simulink model "Complete_HPP_Model_PEM_WIndTurbine"  (R2022a)
settings: Solver=ode4  StartTime=0.0  StopTime=5  FixedStep=1e-6  MaxStep=50e-7  RelTol=1e-3
undefined symbols (not defined in the file or in its folder): DiscIntNeverNeededParam, Ts_Control
libraries: spsMeanLib x9, spsSeriesRLCBranchLib x8, spsIGBTDiodeLib x7, spsVoltageMeasurementLib x6, spsThreePhaseVIMeasurementLib x4, spsDiodeLib x4, spsCurrentMeasurementLib x4, spsMosfetLib x3, spsThreePhaseSeriesRLCBranchLib x2, spsGroundLib x2, spsSawtoothGeneratorLib x2, spsWindTurbineLib x1
(part 1 of 2)
settings Model: Creator=TASOS  LastModifiedBy=nikos
settings DebuggingCC: AlgebraicLoopMsg=none

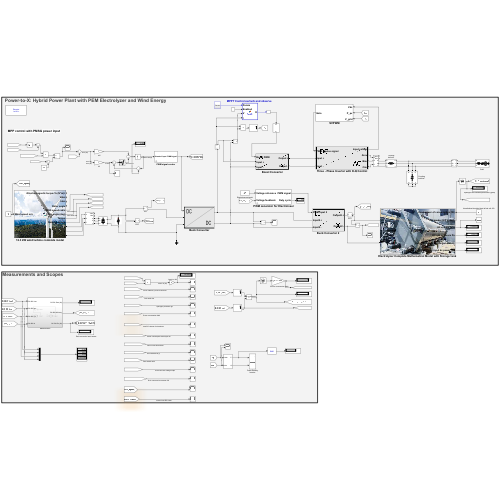
[thumbnail: Simulink's stored preview of the top-level diagram]
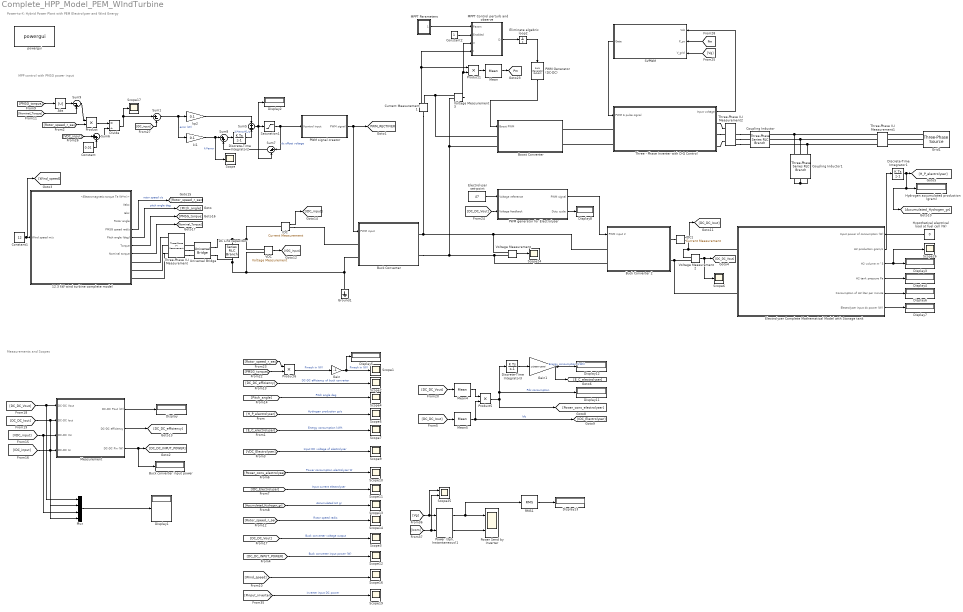
== system Complete_HPP_Model_PEM_WIndTurbine ==
  note: Power-to-X: Hybrid Power Plant with PEM Electrolyzer and Wind Energy
  note: Measurements and Scopes
  note: MPP control with PMSG power input
  12.3 kW wind turbine complete model : Subsystem  mask{Nominal_mechanical_output_power=12.3e3, R=1.3, Base_wind=12}
      mask prompts: Nominal_mechanical_output_power "Nominal_mechanical_output_power (W)"; R "Rotor radiance (m)"; Base_wind "Base_wind (m/s)"
      mask Display: image('$imagefile'); % Use "Edit Image" on toolstrip to change.
  Abs : Abs  SaturateOnIntegerOverflow=off
  Boost Converter : Subsystem
      mask Display: image('$imagefile'); % Use "Edit Image" on toolstrip to change.
  Buck Converter : Subsystem
      mask Display: image('$imagefile'); % Use "Edit Image" on toolstrip to change.
  "Buck Converter 2 " : Subsystem
      mask Display: image('$imagefile'); % Use "Edit Image" on toolstrip to change.
  Buck converter input power : Display
  Constant : Constant  Value=0.01
  Constant1 : Constant  Value=12
  Constant2 : Constant
  Coupling Inductor : spsThreePhaseSeriesRLCBranchLib/Three-Phase Series RLC Branch  LConnTagsString=A|B|C  RConnTagsString=A|B|C  BranchType=L  Resistance=0.09  Inductance=15e-3  Capacitance=1e-6  Measurements=None
  Coupling Inductor1 : spsThreePhaseSeriesRLCBranchLib/Three-Phase Series RLC Branch  LConnTagsString=A|B|C  RConnTagsString=A|B|C  BranchType=C  Resistance=0.09  Inductance=0.28e-3  Capacitance=3e-6  Measurements=None
  Current Measurement1 : spsCurrentMeasurementLib/Current Measurement  PhasorSimulation=off  OutputType=Complex  PSBequivalent=0
  DC Link capacitor : spsSeriesRLCBranchLib/Series RLC Branch  LConnTagsString=__new0  RConnTagsString=__new0  BranchType=C  Resistance=0.005  Inductance=200e-6  SetiL0=off  InitialCurrent=0  Capacitance=3600e-6  Setx0=off  InitialVoltage=150  Measurements=None
  Discrete-Time Integrator1 : DiscreteIntegrator  SampleTime=1e-6  ICPrevOutput=DiscIntNeverNeededParam  ICPrevScaledInput=DiscIntNeverNeededParam
  Discrete-Time Integrator2 : DiscreteIntegrator  InitialCondition=0.01  SampleTime=1e-6  LimitOutput=on  UpperSaturationLimit=0.9  LowerSaturationLimit=0.01  ICPrevOutput=DiscIntNeverNeededParam  ICPrevScaledInput=DiscIntNeverNeededParam
  Discrete-Time Integrator3 : DiscreteIntegrator  SampleTime=1e-6  ICPrevOutput=DiscIntNeverNeededParam  ICPrevScaledInput=DiscIntNeverNeededParam
  Display{,1..8,11..13} (12 alike) : Display
  Divide : Product  Inputs=*/
  Electrolyser set-point : Constant  Value=47
  "Electrolyzer Complete Mathematical Model with Storage tank " : Subsystem
      settings: PortSchema="{\"entries\":[{\"content\":{\"sides\":[{\"content\":{\"connectorIds\":[\"In1\",\"Out1\",\"Out2\",\"Out3\",\"Out4\",\"Out5\"]},\"type\":\"ConnectorPlacement.EquallySpacedRectSide\",\"uuid\":\"586e2a01-0b83-4db1-b05b-c9425d179327\"},{\"content\":{\"connectorIds\":[\"RConn1\",\"RConn2\"],\"side\":\"RIGHT\"},\"type\":\"ConnectorPlacement.EquallySpacedRectSide\",\"uuid\":\"98998693-1c1d-43a0-8265-c06eb7552525\"},{\"content\":{\"connectorIds\":[],\"side\":\"TOP\"},\"type\":\"ConnectorPlacement.EquallySpacedRectSide\",\"uuid\":\"57c96d85-f297-491e-8250-1f4aa33eee63\"}]},\"type\":\"ConnectorPlacement.EquallySpacedConnector\",\"uuid\":\"2efb03bc-2da9-4118-9dbe-8a463fcc009b\"}],\"packageUris\":[\"http://schema.mathworks.com/mf0/Connector/R2020b\"],\"version\":\"1.0\"}"
      mask Display: image('$imagefile'); % Use "Edit Image" on toolstrip to change.
  Eliminate algebric loop2 : UnitDelay  InitialCondition=0.485  SampleTime=Ts_Control  HasFrameUpgradeWarning=on
  Gain : Gain  Gain=-1
  Gain1 : Gain  Gain=1/(3600*1000)
  Grid1 : spsThreePhaseSourceLib/Three-Phase Source  InternalConnection=Yg  VoltagePhases=off  Voltage=400  PhaseAngle=0  Voltage_phases=[25e3 25e3 25e3]/sqrt(3)  PhaseAngles_phases=[0 -120 +120]  Frequency=50  NonIdealSource=on  SpecifyImpedance=on  Resistance=0.8929  Inductance=16.58e-3  ShortCircuitLevel=100e6  BaseVoltage=400  XRratio=10  BusType=swing  Pref=0  Qref=0  Prefabc=[10e3, 10e3, 10e3]  Qrefabc=[0, 0, 0]  Qmin=-inf  Qmax=inf
  Ground1 : spsGroundLib/Ground  LConnTagsString=a
  Hydrogen accumulated production (gram) : Display
  Hypothetical electrical load at fuel cell (W) : Constant  Value=0
  IDC : spsCurrentMeasurementLib/Current Measurement  PhasorSimulation=off  OutputType=Complex  PSBequivalent=0
  IDC1 : spsCurrentMeasurementLib/Current Measurement  PhasorSimulation=off  OutputType=Complex  PSBequivalent=0
  MPPT Parameters : Subsystem
  "MPPT Control perturb and observe  " : MATLAB Function  TreatAsAtomicUnit=on
  Mean : spsMeanLib/Mean  Freq=50  Vinit=0  Ts=0
  Mean4 : spsMeanLib/Mean  Freq=50  Vinit=0  Ts=1e-6
  Mean5 : spsMeanLib/Mean  Freq=50  Vinit=0  Ts=1e-6
  Measurement : Subsystem
  Mux : Mux
  PWM Generator (DC-DC) : spsPWMGeneratorDCDCLib/PWM Generator (DC-DC)  Fsw=10000  Ts=0
  PWM generator for Electrolyser : Subsystem  mask{fs=20000, ki2=0.005, kp2=0.05}
      mask prompts: fs "Switching frequency"; ki2 "ki"; kp2 "kp"
  PWM signal creator : Subsystem  mask{Fs=10e3, Ts=0}
      mask prompts: Fs "Switching frequency"; Ts "Sample time"
  "Power (3ph, Instantaneous)1" : spsPower3phInstantaneousLib/Power (3ph, Instantaneous)
  Power Send by Inverter : Scope  NumInputPorts=2
  Product{,1,5..6} (4 alike) : Product
  RMS1 : spsRMSLib/RMS  TrueRMS=on  Freq=60  RMSInit=120  Ts=0
  SVPWM : Subsystem
  Saturation1 : Saturate  UpperLimit=0.9  LowerLimit=0
  Scope{,1..7,9..14,17,19,24,26} (18 alike) : Scope
  Scope16 : Scope  NumInputPorts=2
  Scope25 : Scope  NumInputPorts=2
  Sum1 : Sum  Inputs=|+-
  Sum5 : Sum
  Sum6 : Sum  Inputs=|++
  Sum7 : Sum  Inputs=|+-
  Sum8 : Sum  Inputs=|++
  Sum9 : Sum  Inputs=|-+
  Three - Phase Inverter with D-Q Control : Subsystem
      mask Display: image('$imagefile'); % Use "Edit Image" on toolstrip to change.
  Three-Phase V-I Measurement : spsThreePhaseVIMeasurementLib/Three-Phase V-I Measurement  VoltageMeasurement=phase-to-ground  SetLabelV=off  LabelV=Vabc  Vpu=off  VpuLL=off  CurrentMeasurement=yes  SetLabelI=off  LabelI=Iabc  Ipu=off  Pbase=100e6  Vbase=500e3  OutputType=Complex  PhasorSimulation=off  PSBequivalent=0
  Three-Phase V-I Measurement1 : spsThreePhaseVIMeasurementLib/Three-Phase V-I Measurement  VoltageMeasurement=phase-to-ground  SetLabelV=on  LabelV=Vg  Vpu=off  VpuLL=off  CurrentMeasurement=yes  SetLabelI=on  LabelI=Icom  Ipu=off  Pbase=100e6  Vbase=500e3  OutputType=Complex  PhasorSimulation=off  PSBequivalent=0
  Three-Phase V-I Measurement2 : spsThreePhaseVIMeasurementLib/Three-Phase V-I Measurement  VoltageMeasurement=phase-to-phase  SetLabelV=off  LabelV=Vg  Vpu=off  VpuLL=off  CurrentMeasurement=yes  SetLabelI=off  LabelI=Icom  Ipu=off  Pbase=100e6  Vbase=500e3  OutputType=Complex  PhasorSimulation=off  PSBequivalent=0
  Universal Bridge : spsUniversalBridgeLib/Universal Bridge  Arms=3  SnubberResistance=1e6  SnubberCapacitance=inf  Device=Diodes  Ron=1e-3  Lon=0  ForwardVoltages="[  0  0  ]"  ForwardVoltage=0  GTOparameters=[ 10e-6 , 20e-6 ]  IGBTparameters=[ 1e-6 , 2e-6 ]  Measurements=None  Measurements_2=None  converterType=Rectifier
  VDC : spsVoltageMeasurementLib/Voltage Measurement  PhasorSimulation=off  OutputType=Complex  PSBequivalent=0
  Voltage Measurement : spsVoltageMeasurementLib/Voltage Measurement  PhasorSimulation=off  OutputType=Complex  PSBequivalent=0
  Voltage Measurement2 : spsVoltageMeasurementLib/Voltage Measurement  PhasorSimulation=off  OutputType=Complex  PSBequivalent=0
  Voltage Measurement3 : spsVoltageMeasurementLib/Voltage Measurement  PhasorSimulation=off  OutputType=Complex  PSBequivalent=0
  ki1 : Gain  Gain=0.1
  kp2 : Gain  Gain=0.1
  powergui : spspowerguiLib/powergui  Priority=1  SimulationMode=Discrete  SampleTime=1e-6  frequency=60  Iterations=50  frequencyindice=0  Pbase=100e6  ErrMax=1e-4  UnitsV=kV  UnitsW=MW  buscounter=0  FunctionMessages=off  echomessages=off  EnableUseOfTLC=off  CurrentSourceSwitches=off  DisableSnubberDevices=off  DisableRonSwitches=off  DisableVfSwitches=off  DisplayEquations=off  AutomaticDiscreteSolvers=off  SolverType=Tustin/Backward Euler (TBE)  Interpol=off  ExternalGateDelay=off  methode=off  Ts=100  x0status=blocks  SPID=on  SwTol=0  HookPort=off  NonlinearTolerance=1e-4  nMaxIteration=100  ContinueOnMaxIteration=off  RestoreLinks=warning  ResistiveCurrentMeasurement=off  Frange=[0:2:500]  Ylog=off  Xlog=on  ShowGrid=off  save=off  variable=ZData  structure=0  ZoomFFT=off  StartTime=0.0  cycles=1  DisplayStyle=1  fundamental=60  FreqAxis=off  MaxFrequency=1000  frequencyindicesteady=1  RmsSteady=1  display=off
  tag scope: PWM_RECTIFIER=global, Pm=global
  wires:
  Mean5/1 -> Product5/2, [IDC_Electrolyser]  "Idc"
  Discrete-Time Integrator3/1 -> Gain1/1
  Gain1/1 -> [E_C_electrolyser], Display12/1  "Energy consumption (kWh)"
  Product5/1 -> Discrete-Time Integrator3/1, Display11/1, [Power_cons_electrolyser]  "Pdc consumption"
  Mean4/1 -> Product5/1
  Product6/1 -> Gain/1  "Pmech in (W)"
  [DC_DC_efficiency] -> Scope2/1  "DC-DC efficiency of buck converter"
  [Pitch_angle] -> Scope4/1  "Pitch angle deg"
  [E_C_electrolyser] -> Scope7/1  "Energy consumption kWh"
  [IDC_Electrolyser] -> Scope11/1  "Input current electrolyser"
  [H_P_electrolyser] -> Scope5/1  "Hydrogen production gr/s"
  [Accumulated_Hydrogen_gr] -> Scope13/1  "Accumulated H2 gr"
  [Power_cons_electrolyser] -> Scope10/1  "Power consumption electrolyser W"
  [VDC_Electrolyser] -> Scope9/1  "Input DC voltage of electrolyser"
  12.3 kW wind turbine complete model/6(Pitch angle (deg)) -> [Pitch_angle]  "pitch angle deg"
  12.3 kW wind turbine complete model/5(PMSG speed rad/s) -> [Rotor_speed_r_sec]  "rotor speed r/s"
  Gain/1 -> Scope1/1, Display5/1  "Pmech in (W)"
  [Rotor_speed_r_sec] -> Scope14/1  "Rotor speed rad/s"
  [DC_DC_Vout] -> Scope3/1  "Buck converter voltage output"
  IDC1/1 -> [DC_DC_Iout]
  Measurement/1(DC-DC Pout (W)) -> Display/1
  [DC_DC_Vout] -> Mux/1, Measurement/1(DC-DC Vout)
  [DC_DC_Iout] -> Mux/2, Measurement/2(DC-DC Iout)
  [VDC_input] -> Mux/3, Measurement/3(DC-DC Vin)
  [IDC_input] -> Mux/4, Measurement/4(DC-DC Iin)
  Measurement/2(DC-DC efficiency) -> [DC_DC_efficiency]
  Measurement/3(DC-DC Pin (W)) -> Buck converter input power/1, [DC_DC_INPUT_POWER]
  [DC_DC_INPUT_POWER] -> Scope12/1  "Buck converter input power (W)"
  Mux/1 -> Display1/1
  [DC_DC_Vout] -> Mean4/1
  [DC_DC_Iout] -> Mean5/1
  [PMSG_torque] -> Product6/2
  [Rotor_speed_r_sec] -> Product6/1
  [Wind_speed] -> Scope16/2
  VDC/1 -> [VDC_input]
  IDC/1 -> [IDC_input]
  Constant1/1 -> 12.3 kW wind turbine complete model/1(Wind speed m/s), [Wind_speed]
  Discrete-Time Integrator1/1 -> [H_P_electrolyser], Hydrogen accumulated production (gram)/1, [Accumulated_Hydrogen_gr]
  "Electrolyzer Complete Mathematical Model with Storage tank "/1(H2 production gram/s) -> Discrete-Time Integrator1/1
  [Pinput_inverter] -> Scope19/1  "inverter input DC power"
  "Electrolyzer Complete Mathematical Model with Storage tank "/2(H2 volume m^3) -> Display3/1, Scope26/1
  "Electrolyzer Complete Mathematical Model with Storage tank "/3(H2 tank pressure Pa) -> Display4/1
  Hypothetical electrical load at fuel cell (W)/1 -> "Electrolyzer Complete Mathematical Model with Storage tank "/1(Input power of consumption (W))
  "Electrolyzer Complete Mathematical Model with Storage tank "/4(Consumption of H2 liter per minute) -> Display6/1
  "Electrolyzer Complete Mathematical Model with Storage tank "/5(Electrolyser input dc power (W)) -> Display7/1
  Voltage Measurement2/1 -> [DC_DC_Vout], Scope6/1
  Electrolyser set-point/1 -> PWM generator for Electrolyser/1(Voltage reference)
  [DC_DC_Vout] -> PWM generator for Electrolyser/2(Voltage feedback)
  PWM generator for Electrolyser/2(Duty cycle) -> Display8/1
  Voltage Measurement/1 -> Scope24/1
  12.3 kW wind turbine complete model/7(Torque) -> [PMSG_torque]
  12.3 kW wind turbine complete model/8(Nominal torque) -> [Nominal_Torque]
  PWM signal creator/1(PWM signal) -> [PWM_RECTIFIER], Buck Converter/1(PWM input)
  PWM generator for Electrolyser/1(PWM signal) -> "Buck Converter 2 "/1(PWM input 2)
  [Pm] -> SVPWM/2(P_pv)
  [Vg] -> SVPWM/3(V_grid)
  MPPT Parameters/1(Param) -> "MPPT Control perturb and observe  "/1(Param)
  Mean/1 -> [Pm]
  Eliminate algebric loop2/1 -> PWM Generator (DC-DC)/1
  "MPPT Control perturb and observe  "/1(D) -> Eliminate algebric loop2/1
  Constant2/1 -> "MPPT Control perturb and observe  "/2(Enabled)
  Product1/1 -> Mean/1
  Current Measurement1/1 -> Product1/1, "MPPT Control perturb and observe  "/4(I)
  Voltage Measurement3/1 -> Product1/2, "MPPT Control perturb and observe  "/3(V)
  PWM Generator (DC-DC)/1 -> Boost Converter/1(Boost PWM)
  Three - Phase Inverter with D-Q Control/1(Input voltage) -> SVPWM/1(Vdc)
  SVPWM/1(Gate) -> Three - Phase Inverter with D-Q Control/1(PWM 6 pulse signal)
  Sum8/1 -> Discrete-Time Integrator2/1
  [IDC_input] -> Sum1/2
  ki1/1 -> Sum8/1, Scope/1  "ki*error"
  Discrete-Time Integrator2/1 -> Sum5/2  "ki*error*1/s"
  Abs/1 -> Sum9/1
  Sum5/1 -> Sum7/2, Display2/1, Saturation1/1
  Divide/1 -> Sum1/1, Scope17/1
  Sum7/1 -> Sum8/2
  Sum9/1 -> Product/1
  Saturation1/1 -> PWM signal creator/1("Vcontrol input "), Sum7/1  "dc offset voltage"
  Product/1 -> Divide/1
  [VDC_input] -> Sum6/1
  Sum1/1 -> kp2/1, ki1/1  "error (W)"
  kp2/1 -> Sum5/1
  [Nominal_Torque] -> Sum9/2
  [Rotor_speed_r_sec] -> Product/2
  Sum6/1 -> Divide/2
  [PMSG_torque] -> Abs/1
  Constant/1 -> Sum6/2
  "Power (3ph, Instantaneous)1"/2 -> Power Send by Inverter/2
  "Power (3ph, Instantaneous)1"/1 -> RMS1/1, Power Send by Inverter/1
  [Vg] -> Scope25/1, "Power (3ph, Instantaneous)1"/1
  [Icom] -> Scope25/2, "Power (3ph, Instantaneous)1"/2
  RMS1/1 -> Display13/1
  connections:
  DC Link capacitor/LConn1 -- IDC/LConn1 -- VDC/LConn1 -- Universal Bridge/RConn1
  Universal Bridge/LConn1 -- Three-Phase V-I Measurement/RConn1
  Three-Phase V-I Measurement/RConn2 -- Universal Bridge/LConn2
  Three-Phase V-I Measurement/RConn3 -- Universal Bridge/LConn3
  Three-Phase V-I Measurement/LConn1 -- 12.3 kW wind turbine complete model/RConn1
  Three-Phase V-I Measurement/LConn2 -- 12.3 kW wind turbine complete model/RConn2
  Three-Phase V-I Measurement/LConn3 -- 12.3 kW wind turbine complete model/RConn3
  IDC1/RConn1 -- "Electrolyzer Complete Mathematical Model with Storage tank "/RConn1 -- Voltage Measurement2/LConn1
  Voltage Measurement/LConn1 -- "Buck Converter 2 "/LConn1 -- Current Measurement1/LConn1 -- Buck Converter/RConn1
  IDC/RConn1 -- Buck Converter/LConn1
  VDC/LConn2 -- Ground1/LConn1 -- Buck Converter/LConn2 -- Universal Bridge/RConn2 -- DC Link capacitor/RConn1
  Voltage Measurement/LConn2 -- Voltage Measurement3/LConn2 -- Boost Converter/LConn2 -- Buck Converter/RConn2 -- "Buck Converter 2 "/LConn2
  Voltage Measurement2/LConn2 -- "Buck Converter 2 "/RConn2 -- "Electrolyzer Complete Mathematical Model with Storage tank "/RConn2
  "Buck Converter 2 "/RConn1 -- IDC1/LConn1
  Current Measurement1/RConn1 -- Boost Converter/LConn1 -- Voltage Measurement3/LConn1
  Grid1/RConn1 -- Three-Phase V-I Measurement1/RConn1
  Three-Phase V-I Measurement1/LConn1 -- Coupling Inductor1/LConn1 -- Coupling Inductor/RConn1
  Grid1/RConn3 -- Three-Phase V-I Measurement1/RConn3
  Grid1/RConn2 -- Three-Phase V-I Measurement1/RConn2
  Three-Phase V-I Measurement1/LConn2 -- Coupling Inductor1/LConn2 -- Coupling Inductor/RConn2
  Three-Phase V-I Measurement1/LConn3 -- Coupling Inductor1/LConn3 -- Coupling Inductor/RConn3
  Coupling Inductor1/RConn1 -- Coupling Inductor1/RConn3 -- Coupling Inductor1/RConn2
  Three - Phase Inverter with D-Q Control/LConn1 -- Boost Converter/RConn1
  Three - Phase Inverter with D-Q Control/LConn2 -- Boost Converter/RConn2
  Three - Phase Inverter with D-Q Control/RConn1 -- Three-Phase V-I Measurement2/LConn1
  Three - Phase Inverter with D-Q Control/RConn2 -- Three-Phase V-I Measurement2/LConn2
  Three - Phase Inverter with D-Q Control/RConn3 -- Three-Phase V-I Measurement2/LConn3
  Three-Phase V-I Measurement2/RConn1 -- Coupling Inductor/LConn1
  Three-Phase V-I Measurement2/RConn2 -- Coupling Inductor/LConn2
  Three-Phase V-I Measurement2/RConn3 -- Coupling Inductor/LConn3

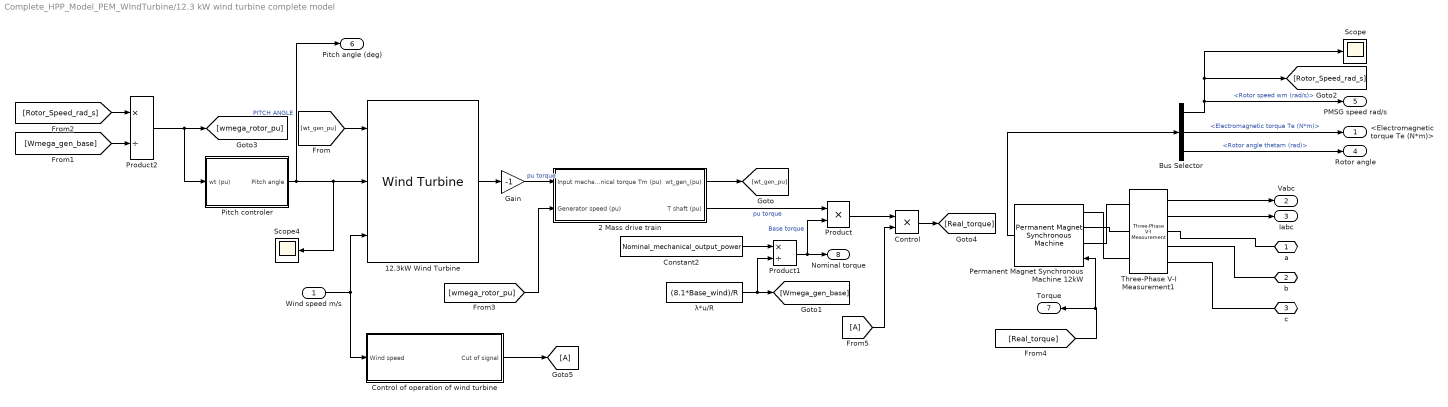
== system Complete_HPP_Model_PEM_WIndTurbine/12.3 kW wind turbine complete model ==
  Wind speed m/s : Inport
  12.3kW Wind Turbine : spsWindTurbineLib/Wind Turbine  Pnom=Nominal_mechanical_output_power  Pelec_base=Nominal_mechanical_output_power/0.9  wind_base=Base_wind  P_wind_base=0.85  speed_nom=1.2  pitch_angle=0  c1_c6="[0.51763          116          0.4            5           21     0.006795]"  cp_nom=0.48  lambda_nom=8.1
      link override Gain: Gain=-1
      settings: SourceProductBaseCode=PS
  2 Mass drive train : Subsystem  mask{H=4, w_base=(8.1*Base_wind)/R, shaft_stiffness=0.3, Ts=1e-6}
      mask prompts: H "Input H"; w_base "Input w base"; shaft_stiffness "Input shaft stiffness"; Ts "Sample time (s)"
  Bus Selector : BusSelector  OutputSignals=Rotor speed wm (rad/s),Electromagnetic torque Te (N*m),Rotor angle thetam (rad)
  Constant2 : Constant  Value=Nominal_mechanical_output_power
  Control : Product
  Control of operation of wind turbine : Subsystem
  From5 : From
  Gain : Gain  Gain=-1
  Goto5 : Goto
  Permanent Magnet Synchronous Machine 12kW : spsPermanentMagnetSynchronousMachineLib/Permanent Magnet Synchronous Machine  NbPhases=3  FluxDistribution=Sinusoidal  RotorType=Salient-pole  MechanicalLoad=Torque Tm  PresetModel=No  ShowDetailedParameters=on  MeasurementBus=off  Resistance=0.425  Inductance=8.5e-3  dqInductances=[0.835e-3, 0.835e-3]  La=1.975e-07  MachineConstant=Flux linkage established by magnets (V.s)  Flux=0.5333  VoltageCst=483.6496  TorqueCst=3.9997  Flat=120  Mechanical=[0.0027 0.000303448 5]  PolePairs=4  InitialConditions=[0,0, 0,0]  InitialConditions5ph=[0 0 0 0 0 0]  RefAngle=90 degrees behind phase A axis (modified Park)  IterativeDiscreteModel=Trapezoidal non iterative  TsBlock=-1  TsPowergui=0
  Pitch controler : Subsystem  mask{Ki=10, Kp=1000}
  Product : Product  Inputs=**
  Product1 : Product  Inputs=*/
  Product2 : Product  Inputs=*/
  Scope : Scope
  Scope4 : Scope
  Three-Phase V-I Measurement1 : spsThreePhaseVIMeasurementLib/Three-Phase V-I Measurement  VoltageMeasurement=phase-to-phase  SetLabelV=off  LabelV=Vabc  Vpu=off  VpuLL=off  CurrentMeasurement=yes  SetLabelI=off  LabelI=Iabc  Ipu=off  Pbase=100e6  Vbase=500e3  OutputType=Complex  PhasorSimulation=off  PSBequivalent=0
  λ*u/R : Constant  Value=(8.1*Base_wind)/R
  a : PMIOPort  Side=Right
  b : PMIOPort  Port=2  Side=Right
  c : PMIOPort  Port=3  Side=Right
  <Electromagnetic torque Te (N*m)> : Outport
  Vabc : Outport  Port=2
  Iabc : Outport  Port=3
  Rotor angle : Outport  Port=4
  PMSG speed rad/s : Outport  Port=5
  Pitch angle (deg) : Outport  Port=6
  Torque : Outport  Port=7
  Nominal torque : Outport  Port=8
  wires:
  Pitch controler/1(Pitch angle) -> Pitch angle (deg)/1, Scope4/1, 12.3kW Wind Turbine/2  "PITCH ANGLE"
  Product2/1 -> [wmega_rotor_pu], Pitch controler/1(wt (pu))
  [wmega_rotor_pu] -> 2 Mass drive train/2(Generator speed (pu))
  Bus Selector/1 -> Scope/1, [Rotor_Speed_rad_s], PMSG speed rad/s/1  "<Rotor speed wm (rad/s)>"
  [Rotor_Speed_rad_s] -> Product2/1
  λ*u/R/1 -> [Wmega_gen_base], Product1/2
  12.3kW Wind Turbine/1 -> Gain/1
  Bus Selector/3 -> Rotor angle/1  "<Rotor angle thetam (rad)>"
  Product1/1 -> Nominal torque/1, Product/2  "Base torque"
  Permanent Magnet Synchronous Machine 12kW/1 -> Bus Selector/1
  [Wmega_gen_base] -> Product2/2
  Constant2/1 -> Product1/1
  Bus Selector/2 -> <Electromagnetic torque Te (N*m)>/1  "<Electromagnetic torque Te (N*m)>"
  Three-Phase V-I Measurement1/1 -> Vabc/1
  Three-Phase V-I Measurement1/2 -> Iabc/1
  Wind speed m/s/1 -> 12.3kW Wind Turbine/3, Control of operation of wind turbine/1(Wind speed)
  Product/1 -> Control/1
  Control/1 -> [Real_torque]
  From5/1 -> Control/2
  Control of operation of wind turbine/1(Cut of signal) -> Goto5/1
  2 Mass drive train/1("wt_gen_(pu) ") -> [wt_gen_pu]
  [wt_gen_pu] -> 12.3kW Wind Turbine/1
  Gain/1 -> 2 Mass drive train/1(Input mechanical torque Tm (pu))  "pu torque"
  2 Mass drive train/2(T shaft (pu)) -> Product/1  "pu torque"
  [Real_torque] -> Permanent Magnet Synchronous Machine 12kW/1, Torque/1
  connections:
  Three-Phase V-I Measurement1/LConn3 -- Permanent Magnet Synchronous Machine 12kW/LConn3
  Three-Phase V-I Measurement1/RConn2 -- b/RConn1
  Three-Phase V-I Measurement1/RConn3 -- c/RConn1
  Three-Phase V-I Measurement1/RConn1 -- a/RConn1
  Three-Phase V-I Measurement1/LConn1 -- Permanent Magnet Synchronous Machine 12kW/LConn1
  Three-Phase V-I Measurement1/LConn2 -- Permanent Magnet Synchronous Machine 12kW/LConn2

== system Complete_HPP_Model_PEM_WIndTurbine/Boost Converter ==
  Boost PWM : Inport
  D : spsDiodeLib/Diode  Ron=0.001  Lon=0  Vf=0.8  IC=0  UseSnubber=0  Rs=inf  Cs=250e-9  Measurements=off
  L : spsSeriesRLCBranchLib/Series RLC Branch  LConnTagsString=__new0  RConnTagsString=__new0  BranchType=L  Resistance=0.001  Inductance=4e-3  SetiL0=off  InitialCurrent=0  Capacitance=1e-6  Setx0=off  InitialVoltage=0  Measurements=None
  S : spsIGBTDiodeLib/IGBT//Diode  Ron=1e-3  Rs=1e5  Cs=inf  Measurements=off
  Output + : PMIOPort  Side=Right
  Output - : PMIOPort  Port=2  Side=Right
  Input + : PMIOPort  Port=3  Side=Left
  Input - : PMIOPort  Port=4  Side=Left
  wires:
  Boost PWM/1 -> S/1
  connections:
  S/RConn1 -- Input -/RConn1 -- Output -/RConn1
  D/LConn1 -- L/RConn1 -- S/LConn1
  Output +/RConn1 -- D/RConn1
  Input +/RConn1 -- L/LConn1

== system Complete_HPP_Model_PEM_WIndTurbine/Buck Converter ==
  note: Buck converter
  note: Vout = D x Vin
      | where: D=Duty cycle
  PWM input : Inport
  Diode1 : spsDiodeLib/Diode  Ron=1e-3  Lon=0  Vf=0.7  IC=0  UseSnubber=off  Rs=1e6  Cs=inf  Measurements=on
  Mosfet1 : spsMosfetLib/Mosfet  Ron=0.01  Lon=0  Rd=1e-3  Vfd=0  IC=0  Rs=1e6  Cs=inf  Measurements=on
  RL : spsSeriesRLCBranchLib/Series RLC Branch  LConnTagsString=__new0  RConnTagsString=__new0  BranchType=RL  Resistance=20e-3  Inductance=1e-3  SetiL0=off  InitialCurrent=0  Capacitance=1e-6  Setx0=off  InitialVoltage=0  Measurements=None
  Series RLC Branch1 : spsSeriesRLCBranchLib/Series RLC Branch  LConnTagsString=__new0  RConnTagsString=__new0  BranchType=C  Resistance=1e-4  Inductance=200e-6  SetiL0=off  InitialCurrent=0  Capacitance=220e-6  Setx0=off  InitialVoltage=150  Measurements=None
  Output + : PMIOPort  Side=Right
  Input + : PMIOPort  Port=2  Side=Left
  Output - : PMIOPort  Port=3  Side=Right
  Input - : PMIOPort  Port=4  Side=Left
  wires:
  PWM input/1 -> Mosfet1/1
  connections:
  Input +/RConn1 -- Mosfet1/LConn1
  Output +/RConn1 -- RL/RConn1 -- Series RLC Branch1/LConn1
  Diode1/RConn1 -- RL/LConn1 -- Mosfet1/RConn1
  Series RLC Branch1/RConn1 -- Input -/RConn1 -- Diode1/LConn1 -- Output -/RConn1

== system Complete_HPP_Model_PEM_WIndTurbine/Buck Converter 2  ==
  note: Buck converter
  note: Vout = D x Vin
      | where: D=Duty cycle
  PWM input 2 : Inport
  Diode : spsDiodeLib/Diode  Ron=0.001  Lon=0  Vf=0.8  IC=0  UseSnubber=off  Rs=500  Cs=250e-9  Measurements=off
  Mosfet1 : spsMosfetLib/Mosfet  Ron=0.01  Lon=0  Rd=1e-3  Vfd=0  IC=0  Rs=1e6  Cs=inf  Measurements=on
  Series RLC Branch : spsSeriesRLCBranchLib/Series RLC Branch  LConnTagsString=__new0  RConnTagsString=__new0  BranchType=RL  Resistance=80e-3  Inductance=161.95e-6  SetiL0=off  InitialCurrent=0  Capacitance=1e-6  Setx0=off  InitialVoltage=0  Measurements=None
  Series RLC Branch1 : spsSeriesRLCBranchLib/Series RLC Branch  LConnTagsString=__new0  RConnTagsString=__new0  BranchType=C  Resistance=1e-4  Inductance=200e-6  SetiL0=off  InitialCurrent=0  Capacitance=2200e-6  Setx0=off  InitialVoltage=150  Measurements=None
  Output2 + : PMIOPort  Side=Right
  Input2 + : PMIOPort  Port=2  Side=Left
  Output2 - : PMIOPort  Port=3  Side=Right
  Input2 - : PMIOPort  Port=4  Side=Left
  wires:
  PWM input 2/1 -> Mosfet1/1
  connections:
  Input2 +/RConn1 -- Mosfet1/LConn1
  Series RLC Branch1/LConn1 -- Output2 +/RConn1 -- Series RLC Branch/RConn1
  Mosfet1/RConn1 -- Series RLC Branch/LConn1 -- Diode/RConn1
  Series RLC Branch1/RConn1 -- Input2 -/RConn1 -- Diode/LConn1 -- Output2 -/RConn1

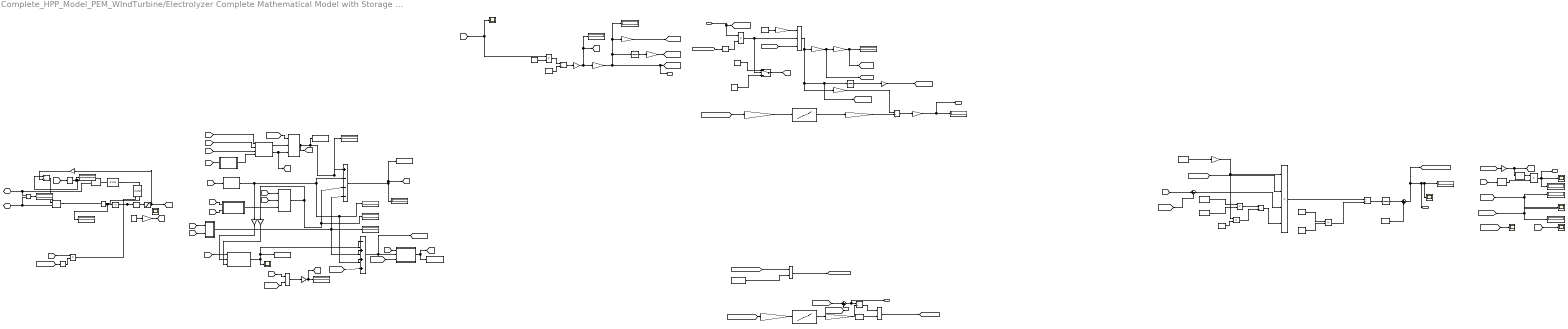
== system Complete_HPP_Model_PEM_WIndTurbine/Electrolyzer Complete Mathematical Model with Storage tank  ==
  note: Measurements
  note: Hydrogen Storage System
  note: Logic Control
  note: Hydrogen Production and Consumption
  note: Steady State - Dynamic Modelling
  note: Hydrogen Production
  note: Hydrogen Consumption
  note: Stops the Load when there is no Hydrogen in the Tank
  note: When Hydrogen Production becomes equal with the Capacity of the Tank, the current cuts off
  Input power of consumption (W) : Inport
  " voltage gain" : Sum  Inputs=|+---
  " voltage gain1" : Sum  Inputs=|-+++
  2F : Constant  Value=2*96485
  Abs : Abs  SaturateOnIntegerOverflow=off
  Concetration losses : Subsystem
  Constant : Constant  Value=475
  Constant2 : Constant
  Constant3 : Constant
  Constant4 : Constant  Value=0
  Constant5 : Constant  Value=1.05
  Controlled Current Source : spsControlledCurrentSourceLib/Controlled Current Source  Initialize=off  Source_Type=DC  Amplitude=0  Phase=0  Frequency=0  Measurements=None
  Controlled Voltage Source1 : spsControlledVoltageSourceLib/Controlled Voltage Source  Initialize=off  Source_Type=DC  Amplitude=0  Phase=0  Frequency=0  Measurements=None
  Current Measurement1 : spsCurrentMeasurementLib/Current Measurement  PhasorSimulation=off  OutputType=Complex  PSBequivalent=0
  Diode1 : spsDiodeLib/Diode  Ron=0.001  Lon=0  Vf=0  IC=0  UseSnubber=0  Rs=10e6  Cs=inf  Measurements=off
  Discrete-Time Integrator : DiscreteIntegrator  SampleTime=1e-6  ICPrevOutput=DiscIntNeverNeededParam  ICPrevScaledInput=DiscIntNeverNeededParam
  Discrete-Time Integrator1 : DiscreteIntegrator  SampleTime=1e-6  ICPrevOutput=DiscIntNeverNeededParam  ICPrevScaledInput=DiscIntNeverNeededParam
  Discrete-Time Integrator2 : DiscreteIntegrator  SampleTime=1e-6  ICPrevOutput=DiscIntNeverNeededParam  ICPrevScaledInput=DiscIntNeverNeededParam
  Display{,1..13} (14 alike) : Display
  Divide{,1..2,4..7} (7 alike) : Product  Inputs=*/
  Divide3 : Product  Inputs=**/
  Dynamic activation losses : Subsystem
  Dynamic temperature model : Subsystem
  Environmental Pressure (Pa) : Constant  Value=101325
  Environmental Temperature (K) : Constant  Value=283.15
  Ernest cell Voltage : Subsystem
  Gain : Gain
  Gain1 : Gain  Gain=1/1000
  Gain2 : Gain  Gain=100
  Gain3 : Gain  Gain=1e-8
  Gain4 : Gain  Gain=100
  Gain5 : Gain  Gain=0.1
  Gram/sec : Gain  Gain=1000
  H2 Molecular Mass (Gram/Mol) : Constant  Value=1.00784
  Hydrogen prod (g/s) : Display
  Hydrogen prod (mol/s) : Display
  Ideal Gas Constant (J/Mol/Kelvin) : Constant  Value=8.314
  Initial Tank Pressure (Pa) : Constant  Value=101325*1.05
  Initial Tank Pressure (Pa)1 : Constant  Value=101325
  J/KMol/Kelvin : Gain  Gain=1e-3
  Kg/minute : Gain  Gain=60
  Mean1 : spsMeanLib/Mean  Freq=50  Vinit=0  Ts=1e-6
  Mean4 : spsMeanLib/Mean  Freq=50  Vinit=0  Ts=1e-6
  Memory : Memory  InitialCondition=6  InheritSampleTime=on
  Memory1 : Memory  InitialCondition=6  InheritSampleTime=on
  Mol/sec : Gain  Gain=1/1.0078
  Mosfet : spsMosfetLib/Mosfet  Ron=0.000001  Lon=0  Rd=0.01  Vfd=0  IC=0  Rs=1000  Cs=inf  Measurements=on
  Multiply : Gain  Gain=-1
  Multiply1 : Gain  Gain=-1
  Multiply2 : Gain  Gain=100
  Ohmic losses : Subsystem
  Oxygen concetration : Subsystem
  Pa : Display
  Partial pressures : Subsystem
  Pascal to psia : Gain  Gain=0.00014503773800722
  Pascal to psia1 : Gain  Gain=0.00014503773800722
  Pressure to hydrogen density for 100F : Lookup_n-D  NumberOfTableDimensions=1  BreakpointsForDimension1=[5 50 100 500 1000 2000 5000 10000]  Table=[0.0017 0.0167 0.0334 0.1646 0.3228 0.6209 1.3875 2.3522]  InternalRulePriority=Speed  RndMeth=Simplest
  Pressure to hydrogen density for 100F1 : Lookup_n-D  NumberOfTableDimensions=1  BreakpointsForDimension1=[5 50 100 500 1000 2000 5000 10000]  Table=[0.0017 0.0167 0.0334 0.1646 0.3228 0.6209 1.3875 2.3522]  InternalRulePriority=Speed  RndMeth=Simplest
  Product{,1..3,5..6,9} (7 alike) : Product
  Product4 : Product  Inputs=4
  Relational Operator1 : RelationalOperator  OutDataTypeStr=boolean  RndMeth=Simplest  InputSameDT=off
  Relational Operator2 : RelationalOperator  Operator=<=  OutDataTypeStr=boolean  RndMeth=Simplest  InputSameDT=off
  Relay : Relay  OnOutputValue=0  OffOutputValue=1
  Relay1 : Relay  OnOutputValue=0  OffOutputValue=1
  Saturation : Saturate  UpperLimit=25  LowerLimit=0
  Saturation pressure H2O : Subsystem
  Scope{,1..7} (8 alike) : Scope
  Steady state activation losses : Subsystem
  Sum1 : Sum  Inputs=|+-
  Sum2 : Sum  Inputs=|++
  Sum3 : Sum  Inputs=|+-
  Switch : Switch  Criteria=u2 > Threshold  Threshold=0.001  SaturateOnIntegerOverflow=off  InputSameDT=off
  Tank Capacity (m3) : Constant  Value=0.85
  To Workspace : ToWorkspace  VariableName=E  SampleTime=-1
  To Workspace1 : ToWorkspace  VariableName=Vsteady  SaveFormat=Timeseries  SampleTime=-1
  To Workspace2 : ToWorkspace  VariableName=Vact_dynamic  SaveFormat=Timeseries  SampleTime=-1
  To Workspace4 : ToWorkspace  VariableName=Cell_Temperature  SaveFormat=Structure With Time  SampleTime=-1
  Total storage capacity m3 : Constant  Value=0.85
  Vol H2 : Constant  Value=22.4
  Voltage Measurement : spsVoltageMeasurementLib/Voltage Measurement  PhasorSimulation=off  OutputType=Complex  PSBequivalent=0
  gram to kg : Gain  Gain=1/1000
  gram/sec to kg/min : Gain  Gain=60/1000
  lb/ft3 to kg/m1 : Gain  Gain=16.01846337396
  lb/ft3 to kg/m3 : Gain  Gain=16.01846337396
  m^3 to litr : Gain  Gain=1000
  moll to grams : Gain  Gain=1.0078
  + : PMIOPort  Tag=PMCPort  Side=Right
  - : PMIOPort  Tag=PMCPort  Port=2  Side=Right
  H2 production gram/s : Outport
  H2 volume m^3 : Outport  Port=2
  H2 tank pressure Pa : Outport  Port=3
  Consumption of H2 liter per minute : Outport  Port=4
  Electrolyser input dc power (W) : Outport  Port=5
  tag scope: Area=global, B=global, CellEff=global, Cell_temperature=global, Consumption2=global, Consumption=global, CurrentLogicControl=global, H2Consume=global, H2ConsumeGpS=global, H2Production_kg=global, HydProduction=global, NH2=global, PowerLogicControl=global, PowerNeeded=global, Production=global, RT_Tank_Pressure_in_Pa=global, Vcell=global, VcellDynamic=global, Vstack=global
  wires:
  [B] -> Product/1
  Relay/1 -> Product/2
  Gain/1 -> [Area]
  [CurrentLogicControl] -> Relay/1
  Constant/1 -> Gain/1
  [Current] -> Steady state activation losses/2(I)
  [Actual_cell_V] -> " voltage gain1"/4
  [PO2] -> Oxygen concetration/2(P_O2)
  [Cell_temperature] -> Saturation pressure H2O/1(T)
  [Current] -> Concetration losses/1(I)
  Oxygen concetration/1(Con_O2) -> Steady state activation losses/3(Con_O2)
  [Cell_temperature] -> Partial pressures/3(T)
  [Current] -> Ohmic losses/1(I)
  [Current] -> Partial pressures/1(I)
  Multiply/1 -> Dynamic activation losses/2(Vcon)
  " voltage gain1"/1 -> Dynamic temperature model/2(Vcell_dynamic), [VcellDynamic]
  Dynamic temperature model/1(T) -> To Workspace4/1, [Cell_temperature]
  [Cell_temperature] -> Ernest cell Voltage/1(T)
  [Current] -> Dynamic temperature model/1(I)
  Multiply1/1 -> Dynamic activation losses/3(V_activation_steady)
  Divide1/1 -> Multiply2/1
  Partial pressures/1(Ph2) -> Ernest cell Voltage/2(P_H2)
  [Vcell] -> Divide1/1
  Ohmic losses/1(nohm) -> " voltage gain1"/2, Display4/1, " voltage gain"/4  "Ohmic voltage"
  [Cell_temperature] -> Ohmic losses/2(T)
  [Area] -> Partial pressures/2(A)
  Ernest cell Voltage/1(E) -> To Workspace/1, Display6/1, " voltage gain"/1, [Actual_cell_V]  "Ernest voltage"
  Steady state activation losses/1(n_act) -> Display8/1, " voltage gain"/3, Multiply1/1  "Activation voltage"
  Saturation pressure H2O/1(Psat_H2O) -> Partial pressures/4(ph2osat)
  " voltage gain"/1 -> [Vcell], To Workspace1/1, Display/1
  [Cell_temperature] -> Oxygen concetration/1(T)
  [Actual_cell_V] -> Dynamic temperature model/3(E)
  Partial pressures/2(Po2) -> Ernest cell Voltage/3(P_O2), [PO2]
  Dynamic activation losses/1(vact) -> Scope/1, " voltage gain1"/1, To Workspace2/1  "Dynamic activation voltage"
  [Actual_cell_V] -> Divide1/2
  [Current] -> Dynamic activation losses/1(I)
  Multiply2/1 -> [CellEff], Display5/1
  Concetration losses/1(conc losses) -> " voltage gain1"/3, Display7/1, " voltage gain"/2, Multiply/1  "concetration voltage"
  [Cell_temperature] -> Steady state activation losses/1(T)
  Gain1/1 -> [Consumption]
  Divide3/1 -> [Consumption2], Discrete-Time Integrator1/1, Kg/minute/1, Gram/sec/1
  Discrete-Time Integrator1/1 -> Gain1/1
  Switch/1 -> [B]
  Constant3/1 -> Switch/3
  Constant4/1 -> Switch/1
  Constant5/1 -> Gain3/1
  [PowerLogicControl] -> Relay1/1
  Mol/sec/1 -> [H2Consume], Display9/1
  Product1/1 -> Switch/2, Divide3/2
  Gram/sec/1 -> [H2ConsumeGpS], Mol/sec/1
  Kg/minute/1 -> Divide2/1
  Pressure to hydrogen density for 100F/1 -> lb/ft3 to kg/m3/1  "lbm/ft^3"
  Gain3/1 -> Divide3/1
  Divide2/1 -> m^3 to litr/1
  [RT_Tank_Pressure_in_Pa] -> Pascal to psia/1
  lb/ft3 to kg/m3/1 -> Divide2/2
  [VcellDynamic] -> Divide3/3
  m^3 to litr/1 -> Consumption of H2 liter per minute/1, Display10/1  "liter per minute"
  Relay1/1 -> Product1/2
  Pascal to psia/1 -> Pressure to hydrogen density for 100F/1
  gram/sec to kg/min/1 -> [Production]
  moll to grams/1 -> Hydrogen prod (g/s)/1, gram/sec to kg/min/1, Discrete-Time Integrator2/1, H2 production gram/s/1, [HydProduction]
  gram to kg/1 -> [H2Production_kg]
  Discrete-Time Integrator2/1 -> gram to kg/1
  2F/1 -> Divide/2
  Product2/1 -> Divide/1
  [Current] -> Scope2/1, Product2/1
  Gain2/1 -> [NH2], Hydrogen prod (mol/s)/1, moll to grams/1
  Divide/1 -> Gain2/1
  Constant2/1 -> Product2/2
  [H2Production_kg] -> Sum1/1
  Sum1/1 -> H2 volume m^3/1, Divide4/1
  [Consumption] -> Sum1/2
  Relational Operator1/1 -> [CurrentLogicControl]
  Relational Operator2/1 -> [PowerLogicControl]
  Total storage capacity m3/1 -> Relational Operator1/2
  Divide4/1 -> Relational Operator1/1
  lb/ft3 to kg/m1/1 -> Divide4/2
  Pascal to psia1/1 -> Pressure to hydrogen density for 100F1/1
  Pressure to hydrogen density for 100F1/1 -> lb/ft3 to kg/m1/1  "lbm/ft^3"
  [RT_Tank_Pressure_in_Pa] -> Pascal to psia1/1
  Initial Tank Pressure (Pa)/1 -> Relational Operator2/2
  [RT_Tank_Pressure_in_Pa] -> Relational Operator2/1
  [H2Consume] -> Sum3/2
  J/KMol/Kelvin/1 -> Product4/1, Product3/1
  H2 Molecular Mass (Gram/Mol)/1 -> Product5/1
  [Cell_temperature] -> Product4/2
  Divide5/1 -> Product4/4
  Product4/1 -> Divide6/1
  Divide6/1 -> Discrete-Time Integrator/1
  Product5/1 -> Divide6/2
  Initial Tank Pressure (Pa)1/1 -> Sum2/2  "1 atm"
  Sum3/1 -> Product4/3
  Sum2/1 -> [RT_Tank_Pressure_in_Pa], H2 tank pressure Pa/1, Scope1/1, Pa/1
  Vol H2/1 -> Product6/2
  [NH2] -> Sum3/1
  Discrete-Time Integrator/1 -> Sum2/1
  Environmental Temperature (K)/1 -> Product3/2
  Tank Capacity (m3)/1 -> Product5/2
  Product6/1 -> Divide5/1
  Environmental Pressure (Pa)/1 -> Product6/1
  Ideal Gas Constant (J/Mol/Kelvin)/1 -> J/KMol/Kelvin/1
  Product3/1 -> Divide5/2
  [Production] -> Display11/1, Scope4/1
  [VcellDynamic] -> Gain4/1
  Gain4/1 -> [Vstack], Mean4/1
  Product9/1 -> Electrolyser input dc power (W)/1, Display13/1, Scope3/1
  [CellEff] -> Scope5/1
  [Cell_temperature] -> Scope7/1
  [Consumption2] -> Display12/1
  Product/1 -> Mosfet/1
  Input power of consumption (W)/1 -> [PowerNeeded], Product1/1
  Mean4/1 -> Product9/1
  [Current] -> Mean1/1
  Mean1/1 -> Product9/2
  Memory/1 -> Saturation/1
  Current Measurement1/1 -> Display3/1, Abs/1  "Input current"
  Memory1/1 -> Display1/1, Divide7/1, Controlled Voltage Source1/1
  [Vstack] -> Memory1/1
  Abs/1 -> Memory/1
  Divide7/1 -> Controlled Current Source/1
  Saturation/1 -> [Current], Gain5/1
  Gain5/1 -> Divide7/2
  Voltage Measurement/1 -> Display2/1
  connections:
  Controlled Voltage Source1/LConn1 -- Voltage Measurement/LConn1 -- -/RConn1
  Diode1/LConn1 -- Mosfet/RConn1
  Diode1/RConn1 -- Controlled Voltage Source1/RConn1
  Controlled Current Source/LConn1 -- Voltage Measurement/LConn2 -- +/RConn1
  Controlled Current Source/RConn1 -- Current Measurement1/LConn1
  Mosfet/LConn1 -- Current Measurement1/RConn1

== system Complete_HPP_Model_PEM_WIndTurbine/MPPT Parameters ==
  note: Upper limit for D (Dmax)
  note: Increment value (DeltaD)
  note: Initial value for D output (Dinit)
  note: Lower limit for D (Dmax)
  note: Parameters for Perturb and Observe Algorithm:
  Iph_ : Constant  Value=0.62
  Iph_1 : Constant  Value=0.8
  Iph_2 : Constant  Value=0.2
  Iph_3 : Constant  Value=2e-3
  Mux : Mux
  Param : Outport
  wires:
  Iph_/1 -> Mux/1
  Iph_1/1 -> Mux/2
  Iph_2/1 -> Mux/3
  Iph_3/1 -> Mux/4
  Mux/1 -> Param/1

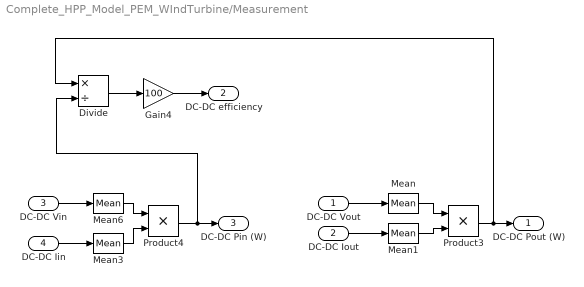
== system Complete_HPP_Model_PEM_WIndTurbine/Measurement ==
  DC-DC Vout : Inport
  DC-DC Iout : Inport  Port=2
  DC-DC Vin : Inport  Port=3
  DC-DC Iin : Inport  Port=4
  Divide : Product  Inputs=*/
  Gain4 : Gain  Gain=100
  Mean{,1,3,6} (4 alike) : spsMeanLib/Mean  Freq=50  Vinit=0  Ts=1e-6
  Product3 : Product
  Product4 : Product
  DC-DC Pout (W) : Outport
  DC-DC efficiency : Outport  Port=2
  DC-DC Pin (W) : Outport  Port=3
  wires:
  Mean/1 -> Product3/1
  Divide/1 -> Gain4/1
  Mean1/1 -> Product3/2
  Product3/1 -> Divide/1, DC-DC Pout (W)/1
  Gain4/1 -> DC-DC efficiency/1
  Product4/1 -> Divide/2, DC-DC Pin (W)/1
  Mean3/1 -> Product4/2
  Mean6/1 -> Product4/1
  DC-DC Vout/1 -> Mean/1
  DC-DC Iout/1 -> Mean1/1
  DC-DC Vin/1 -> Mean6/1
  DC-DC Iin/1 -> Mean3/1

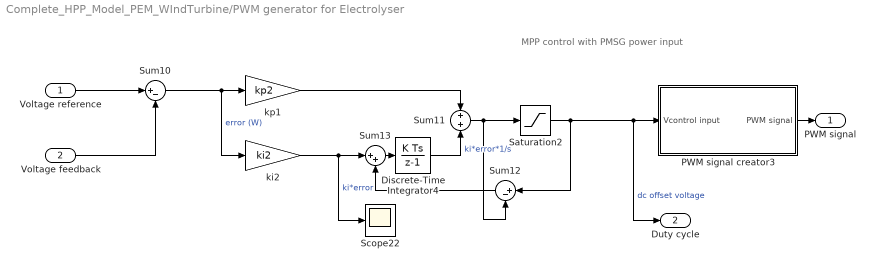
== system Complete_HPP_Model_PEM_WIndTurbine/PWM generator for Electrolyser ==
  note: MPP control with PMSG power input
  Voltage reference : Inport
  Voltage feedback : Inport  Port=2
  Discrete-Time Integrator4 : DiscreteIntegrator  InitialCondition=0.01  SampleTime=1e-6  LimitOutput=on  UpperSaturationLimit=0.9  LowerSaturationLimit=0.01  ICPrevOutput=DiscIntNeverNeededParam  ICPrevScaledInput=DiscIntNeverNeededParam
  PWM signal creator3 : Subsystem  mask{Fs=fs, Ts=0}
      mask prompts: Fs "Switching frequency"; Ts "Sample time"
  Saturation2 : Saturate  UpperLimit=0.95  LowerLimit=0.01
  Scope22 : Scope
  Sum10 : Sum  Inputs=|+-
  Sum11 : Sum
  Sum12 : Sum  Inputs=|+-
  Sum13 : Sum  Inputs=|++
  ki2 : Gain  Gain=ki2
  kp1 : Gain  Gain=kp2
  PWM signal : Outport
  Duty cycle : Outport  Port=2
  wires:
  Saturation2/1 -> Sum12/1, Duty cycle/1, PWM signal creator3/1("Vcontrol input ")  "dc offset voltage"
  Sum13/1 -> Discrete-Time Integrator4/1
  Sum10/1 -> kp1/1, ki2/1  "error (W)"
  Discrete-Time Integrator4/1 -> Sum11/2  "ki*error*1/s"
  kp1/1 -> Sum11/1
  Sum12/1 -> Sum13/2
  Sum11/1 -> Saturation2/1, Sum12/2
  ki2/1 -> Sum13/1, Scope22/1  "ki*error"
  Voltage reference/1 -> Sum10/1
  PWM signal creator3/1(PWM signal) -> PWM signal/1
  Voltage feedback/1 -> Sum10/2

== system Complete_HPP_Model_PEM_WIndTurbine/PWM signal creator ==
  "Vcontrol input " : Inport
  1V peak to peak : spsSawtoothGeneratorLib/Sawtooth Generator  Freq=Fs  Phase=0  Ts=Ts
  Add dc offset : Constant
  Divide1 : Product  Inputs=*/
  Relational Operator : RelationalOperator  Operator=<=  OutDataTypeStr=boolean  RndMeth=Simplest  InputSameDT=off
  Scope11 : Scope  NumInputPorts=3
  Sum1 : Sum  Inputs=|++
  make 0-1V : Constant  Value=2
  PWM signal : Outport
  wires:
  Sum1/1 -> Divide1/1
  Divide1/1 -> Scope11/1, Relational Operator/1  "sawtooth"
  Relational Operator/1 -> PWM signal/1, Scope11/3  "pwm"
  1V peak to peak/1 -> Sum1/1
  "Vcontrol input "/1 -> Relational Operator/2, Scope11/2  "vcontrol"
  make 0-1V/1 -> Divide1/2
  Add dc offset/1 -> Sum1/2

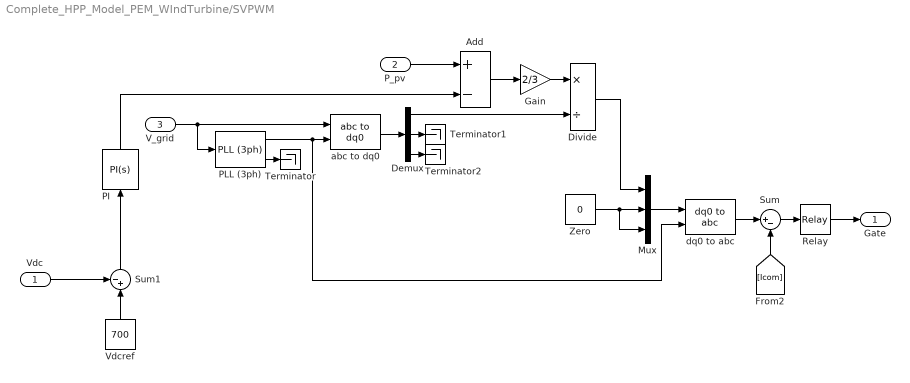
== system Complete_HPP_Model_PEM_WIndTurbine/SVPWM ==
  Vdc : Inport
  P_pv : Inport  Port=2
  V_grid : Inport  Port=3
  Add : Sum  Inputs=+-
  Demux : Demux  Outputs=3
  Divide : Product  Inputs=*/
  Gain : Gain  Gain=2/3
  Mux : Mux  Inputs=3
  PI : slpidlib/PID Controller  Controller=PI  Form=Parallel  TimeDomain=Continuous-time  UseExternalTs=off  SampleTime=-1  IntegratorMethod=Forward Euler  FilterMethod=Forward Euler  ControllerParametersSource=internal  P=112  I=735  UseKiTs=off  D=0  N=100  UseFilter=on  TunerSelectOption=Transfer Function Based (PID Tuner App)  InitialConditionSource=internal  InitialConditionForIntegrator=0  InitialConditionForFilter=0  DifferentiatorICPrevScaledInput=0  ExternalReset=none  TrackingMode=off  Kt=1  LimitOutput=off  SatLimitsSource=internal  UpperSaturationLimit=inf  LowerSaturationLimit=-inf  LinearizeAsGain=on  AntiWindupMode=none  Kb=1  POutMin=[]  POutMax=[]  IOutMin=[]  IOutMax=[]  DOutMin=[]  DOutMax=[]  NOutMin=[]  NOutMax=[]  SumOutMin=[]  SumOutMax=[]  SaturationOutMin=[]  SaturationOutMax=[]  PParamMin=[]  PParamMax=[]  IParamMin=[]  IParamMax=[]  DParamMin=[]  DParamMax=[]  NParamMin=[]  NParamMax=[]  KbParamMin=[]  KbParamMax=[]  KtParamMin=[]  KtParamMax=[]  KbOutMin=[]  KbOutMax=[]  KtOutMin=[]  KtOutMax=[]  IntegratorOutMin=[]  IntegratorOutMax=[]  FilterOutMin=[]  FilterOutMax=[]  SumI1OutMin=[]  SumI1OutMax=[]  SumI2OutMin=[]  SumI2OutMax=[]  SumI3OutMin=[]  SumI3OutMax=[]  SumI4OutMin=[]  SumI4OutMax=[]  SumDOutMin=[]  SumDOutMax=[]  DifferentiatorOutMin=[]  DifferentiatorOutMax=[]  FilterDiffOutCoefMin=[]  FilterDiffOutCoefMax=[]  ReciprocalOutMin=[]  ReciprocalOutMax=[]  SumDenOutMin=[]  SumDenOutMax=[]  SumNumOutMin=[]  SumNumOutMax=[]  DivideOutMin=[]  DivideOutMax=[]  UdiffTsProdOutMin=[]  UdiffTsProdOutMax=[]  NTsProdOutMin=[]  NTsProdOutMax=[]  UintegralTsProdOutMin=[]  UintegralTsProdOutMax=[]  UngainTsProdOutMin=[]  UngainTsProdOutMax=[]  IntegratorContinuousStateAttributes=''  IntegratorStateMustResolveToSignalObject=off  IntegratorRTWStateStorageClass=Auto  FilterContinuousStateAttributes=''  FilterStateMustResolveToSignalObject=off  FilterRTWStateStorageClass=Auto  ParallelPVariant=InternalParameters  IdealPVariant=Disabled  IVariant=InternalParameters  DVariant=Disabled  IntegratorVariant=Continuous  SatVariant=Disabled  AWVariant=Passthrough  PCopyVariant=Disabled  TRVariant=Disabled  FdbkBlocksVariant=Forward  IdealPFdbkVariant=Disabled  SatFdbkVariant=Disabled  DerivativeFilterVariant=Disabled  NVariant=Disabled  NCopyVariant=Disabled_SignalSpec  FilterICVariant=Disabled  IntegratorICVariant=InternalICs  ExternalResetVariant=Disabled  TRSumVariant=Passthrough  SumFdbkVariant=Disabled  SumVariant=Sum_PI  TsampFilterVariant=InternalTs  TsampNgainVariant=Passthrough  TsampIntegralVariant=Passthrough  ExternalSaturationOutDataTypeStr=Inherit: Same as second input  aMode=0
  PLL (3ph) : spsPLL3phLib/PLL (3ph)  Fmin=45  Par_Init=[0, 60]  ParK=[180, 3200, 1]  TcD=1e-4  MaxRateChangeFreq=12  FilterCutOffFreq=25  Ts=0  AGC=on
  Relay : Relay  OnSwitchValue=0.1  OffSwitchValue=-0.1
  Sum : Sum  Inputs=|+-
  Sum1 : Sum  Inputs=-+|
  Terminator : Terminator
  Terminator1 : Terminator
  Terminator2 : Terminator
  Vdcref : Constant  Value=700
  Zero : Constant  Value=0
  abc to dq0 : spsabctodq0Lib/abc to dq0  Alignment=90 degrees behind phase A axis
  dq0 to abc : spsdq0toabcLib/dq0 to abc  Alignment=90 degrees behind phase A axis
  Gate : Outport
  wires:
  Add/1 -> Gain/1
  Sum1/1 -> PI/1
  Vdc/1 -> Sum1/1
  dq0 to abc/1 -> Sum/1
  PI/1 -> Add/2
  Relay/1 -> Gate/1
  Mux/1 -> dq0 to abc/1
  abc to dq0/1 -> Demux/1
  P_pv/1 -> Add/1
  Gain/1 -> Divide/1
  V_grid/1 -> abc to dq0/1, PLL (3ph)/1
  Divide/1 -> Mux/1
  PLL (3ph)/1 -> Terminator/1
  Zero/1 -> Mux/3, Mux/2
  Demux/2 -> Terminator1/1
  Demux/3 -> Terminator2/1
  Demux/1 -> Divide/2
  PLL (3ph)/2 -> dq0 to abc/2, abc to dq0/2
  Sum/1 -> Relay/1
  [Icom] -> Sum/2
  Vdcref/1 -> Sum1/2

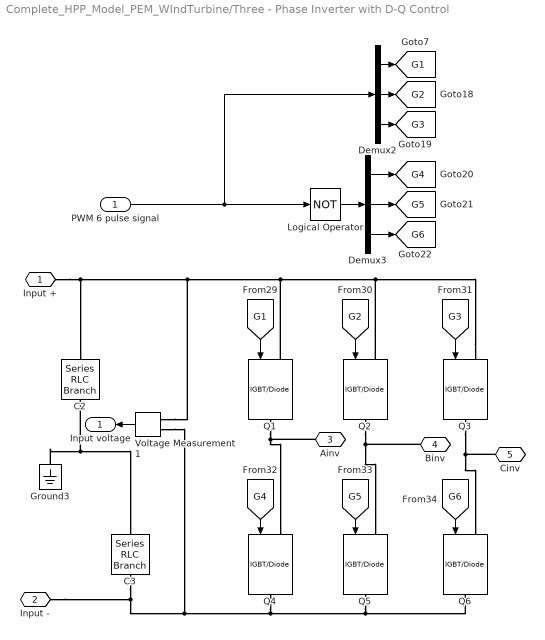
== system Complete_HPP_Model_PEM_WIndTurbine/Three - Phase Inverter with D-Q Control ==
  PWM 6 pulse signal : Inport
  C2 : spsSeriesRLCBranchLib/Series RLC Branch  LConnTagsString=__new0  RConnTagsString=__new0  BranchType=C  Resistance=1  Inductance=1e-3  SetiL0=off  InitialCurrent=0  Capacitance=4700e-6  Setx0=on  InitialVoltage=350  Measurements=None
  C3 : spsSeriesRLCBranchLib/Series RLC Branch  LConnTagsString=__new0  RConnTagsString=__new0  BranchType=C  Resistance=1  Inductance=1e-3  SetiL0=off  InitialCurrent=0  Capacitance=4700e-6  Setx0=on  InitialVoltage=350  Measurements=None
  Demux2 : Demux  Outputs=3
  Demux3 : Demux  Outputs=3
  Ground3 : spsGroundLib/Ground  LConnTagsString=a
  Logical Operator : Logic  Operator=NOT  IconShape=distinctive  AllPortsSameDT=off  OutDataTypeStr=boolean
  Q{1..6} (6 alike) : spsIGBTDiodeLib/IGBT//Diode  Ron=1e-3  Rs=1e5  Cs=inf  Measurements=off
  Voltage Measurement1 : spsVoltageMeasurementLib/Voltage Measurement  PhasorSimulation=off  OutputType=Complex  PSBequivalent=0
  Input + : PMIOPort  Side=Left
  Input - : PMIOPort  Port=2  Side=Left
  "Ainv " : PMIOPort  Port=3  Side=Right
  Binv : PMIOPort  Port=4  Side=Right
  Cinv : PMIOPort  Port=5  Side=Right
  Input voltage : Outport
  tag scope: G1=global, G2=global, G3=global, G4=global, G5=global, G6=global
  wires:
  [G4] -> Q4/1
  [G2] -> Q2/1
  Demux3/3 -> [G6]
  [G5] -> Q5/1
  Demux2/3 -> [G3]
  [G1] -> Q1/1
  Logical Operator/1 -> Demux3/1
  [G6] -> Q6/1
  Demux2/2 -> [G2]
  [G3] -> Q3/1
  Demux3/2 -> [G5]
  Voltage Measurement1/1 -> Input voltage/1
  Demux3/1 -> [G4]
  Demux2/1 -> [G1]
  PWM 6 pulse signal/1 -> Demux2/1, Logical Operator/1
  connections:
  Q3/LConn1 -- Input +/RConn1 -- C2/LConn1 -- Voltage Measurement1/LConn1 -- Q1/LConn1 -- Q2/LConn1
  Q2/RConn1 -- Binv/RConn1 -- Q5/LConn1
  Q1/RConn1 -- "Ainv "/RConn1 -- Q4/LConn1
  Voltage Measurement1/LConn2 -- Input -/RConn1 -- C3/RConn1 -- Q6/RConn1 -- Q5/RConn1 -- Q4/RConn1
  Q3/RConn1 -- Cinv/RConn1 -- Q6/LConn1
  C2/RConn1 -- C3/LConn1 -- Ground3/LConn1

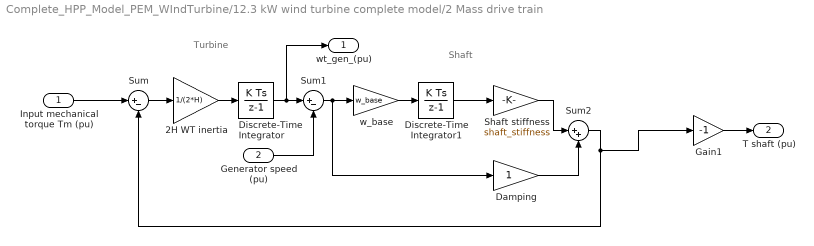
== system Complete_HPP_Model_PEM_WIndTurbine/12.3 kW wind turbine complete model/2 Mass drive train ==
  note: Shaft
  note: Turbine
  Input mechanical torque Tm (pu) : Inport
  Generator speed (pu) : Inport  Port=2
  2H WT inertia : Gain  Gain=1/(2*H)
  Damping : Gain
  Discrete-Time Integrator : DiscreteIntegrator  InitialCondition=1  SampleTime=Ts  ICPrevOutput=DiscIntNeverNeededParam  ICPrevScaledInput=DiscIntNeverNeededParam
  Discrete-Time Integrator1 : DiscreteIntegrator  InitialCondition=1/shaft_stiffness  SampleTime=Ts  ICPrevOutput=DiscIntNeverNeededParam  ICPrevScaledInput=DiscIntNeverNeededParam
  Gain1 : Gain  Gain=-1
  Shaft stiffness : Gain  Gain=shaft_stiffness
  Sum : Sum  Inputs=|+-
  Sum1 : Sum  Inputs=|+-
  Sum2 : Sum  Inputs=|++
  w_base : Gain  Gain=w_base
  "wt_gen_(pu) " : Outport
  T shaft (pu) : Outport  Port=2
  wires:
  Damping/1 -> Sum2/2
  2H WT inertia/1 -> Discrete-Time Integrator/1
  Sum1/1 -> Damping/1, w_base/1
  Generator speed (pu)/1 -> Sum1/2
  Sum/1 -> 2H WT inertia/1
  Input mechanical torque Tm (pu)/1 -> Sum/1
  Discrete-Time Integrator1/1 -> Shaft stiffness/1
  Shaft stiffness/1 -> Sum2/1
  w_base/1 -> Discrete-Time Integrator1/1
  Discrete-Time Integrator/1 -> "wt_gen_(pu) "/1, Sum1/1
  Sum2/1 -> Gain1/1, Sum/2
  Gain1/1 -> T shaft (pu)/1

== system Complete_HPP_Model_PEM_WIndTurbine/12.3 kW wind turbine complete model/Control of operation of wind turbine ==
  Wind speed : Inport
  Constant : Constant  Value=0
  Constant1 : Constant
  Cutt off on wind speed : MATLAB Function  TreatAsAtomicUnit=on
  Display : Display
  Switch : Switch  Criteria=u2 > Threshold  SaturateOnIntegerOverflow=off  InputSameDT=off
  Cut of signal : Outport
  wires:
  Wind speed/1 -> Cutt off on wind speed/1(u)
  Switch/1 -> Cut of signal/1
  Cutt off on wind speed/1(y) -> Switch/2, Display/1
  Constant1/1 -> Switch/3
  Constant/1 -> Switch/1

== system Complete_HPP_Model_PEM_WIndTurbine/12.3 kW wind turbine complete model/Pitch controler ==
  wt (pu) : Inport
  Constant : Constant  Value=1.2
  Discrete-Time Integrator : DiscreteIntegrator  InitialCondition=5  SampleTime=1e-6  ICPrevOutput=DiscIntNeverNeededParam  ICPrevScaledInput=DiscIntNeverNeededParam
  Rate Limiter : RateLimiter  RisingSlewLimit=100  FallingSlewLimit=-100  SampleTimeMode=inherited
  Saturation : Saturate  UpperLimit=45  LowerLimit=0
  Scope : Scope
  Sum : Sum  Inputs=|+-
  Sum2 : Sum
  Sum4 : Sum  Inputs=|++
  ki : Gain  Gain=Ki
  kp : Gain  Gain=Kp
  Pitch angle : Outport
  wires:
  wt (pu)/1 -> Sum/1
  Constant/1 -> Sum/2
  Sum4/1 -> Discrete-Time Integrator/1  "ki*error"
  ki/1 -> Sum4/1
  kp/1 -> Sum2/1
  Sum/1 -> kp/1, ki/1  "error (W)"
  Discrete-Time Integrator/1 -> Sum2/2  "ki*error*1/s"
  Sum2/1 -> Saturation/1
  Saturation/1 -> Rate Limiter/1
  Rate Limiter/1 -> Scope/1, Pitch angle/1

== system Complete_HPP_Model_PEM_WIndTurbine/Electrolyzer Complete Mathematical Model with Storage tank /Concetration losses ==
  I : Inport
  . : Sum  Inputs=|-+
  B : Constant  Value=0.016
  Constant3 : Constant
  Divide2 : Product  Inputs=*/
  Exp : Math  Operator=log
  Product : Product
  limiting current : Constant  Value=25.1
  conc losses : Outport
  wires:
  Exp/1 -> Product/1
  Product/1 -> conc losses/1
  Constant3/1 -> ./2
  B/1 -> Product/2
  Divide2/1 -> ./1
  limiting current/1 -> Divide2/2
  I/1 -> Divide2/1
  ./1 -> Exp/1
